simulink model "lab3DTSys"  (Simulink 8.9)
settings: Solver=ode45  StartTime=0.0  StopTime=100.0  RelTol=1e-3  AbsTol=1e-6
settings Model: SuppressorTable=22 serialization::archive 11 0 6 0 0 0 11 0  Creator=vise  LastModifiedBy=dangd  ExtModeTrigMode=oneshot  ExtModeArmWhenConnect=off
settings DataIOCC: LimitDataPoints=off
settings OptimizationCC: BlockReduction=off  BooleanDataType=off  ExpressionDepthLimit=2147483647  InitFltsAndDblsToZero=on
settings DebuggingCC: SaveWithParameterizedLinksMsg=none  SignalResolutionControl=TryResolveAllWithWarning  MultiTaskDSMMsg=warning  MultiTaskCondExecSysMsg=none
settings HardwareCC: TargetUnknown=on
settings RTWCC: TemplateMakefile=grt_unix.tmf
settings GRTTargetCC: GeneratePreprocessorConditionals=Use local settings

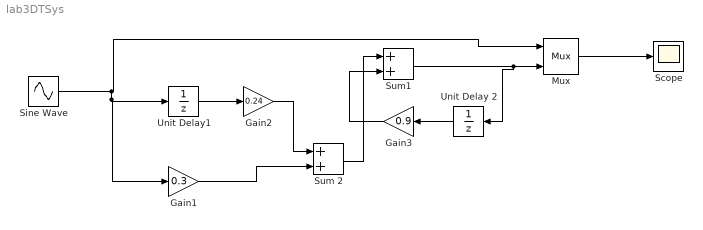
== system lab3DTSys ==
  Gain1 : Gain  Gain=0.3  SaturateOnIntegerOverflow=on  OutDataTypeStr=Inherit: Same as input  ParamDataTypeStr=Inherit: Same as input
  Gain2 : Gain  Gain=0.24  SaturateOnIntegerOverflow=on  OutDataTypeStr=Inherit: Same as input  ParamDataTypeStr=Inherit: Same as input
  Gain3 : Gain  Gain=0.9  SaturateOnIntegerOverflow=on  OutDataTypeStr=Inherit: Same as input  ParamDataTypeStr=Inherit: Same as input
  Mux : Mux  Inputs=2
  Scope : Scope
  Sine Wave : Sin  Frequency=pi/4  SampleTime=1
  Sum 2 : Sum  SaturateOnIntegerOverflow=on  InputSameDT=on  OutDataTypeStr=Inherit: Same as first input
  Sum1 : Sum  SaturateOnIntegerOverflow=on  InputSameDT=on  OutDataTypeStr=Inherit: Same as first input
  Unit Delay 2 : UnitDelay
  Unit Delay1 : UnitDelay
  wires:
  Mux/1 -> Scope/1
  Unit Delay1/1 -> Gain2/1
  Gain1/1 -> Sum 2/2
  Gain2/1 -> Sum 2/1
  Unit Delay 2/1 -> Gain3/1
  Sum 2/1 -> Sum1/1
  Gain3/1 -> Sum1/2
  Sum1/1 -> Unit Delay 2/1, Mux/2
  Sine Wave/1 -> Gain1/1, Unit Delay1/1, Mux/1
